simulink model "equivalence"  (R2021b)
settings: Solver=VariableStepAuto  StartTime=0.0  StopTime=10.0  RelTol=1e-3
settings Model: Creator=user  LastModifiedBy=wangzixuan

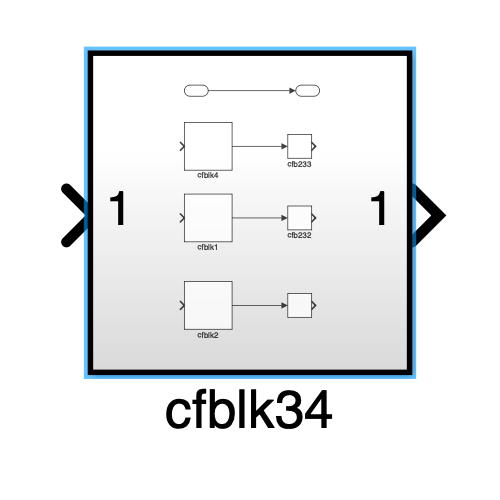
[thumbnail: Simulink's stored preview of the top-level diagram]
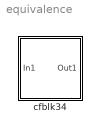
== system equivalence ==
  cfblk34 : Subsystem  TreatAsAtomicUnit=on

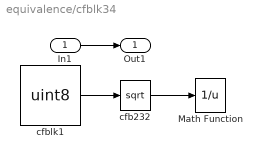
== system equivalence/cfblk34 ==
  In1 : Inport
  Math Function : Math  Operator=reciprocal  SaturateOnIntegerOverflow=on
  cfb232 : Sqrt  SaturateOnIntegerOverflow=on
  cfblk1 : DataTypeConversion  OutDataTypeStr=uint8
  Out1 : Outport
  wires:
  In1/1 -> Out1/1
  cfblk1/1 -> cfb232/1
  cfb232/1 -> Math Function/1
